simulink model "wahadlo3"  (R2018a)
settings: Solver=VariableStepAuto  StartTime=0.0  StopTime=100.0  RelTol=1e-3
settings Model: Creator=Koala  LastModifiedBy=Koala

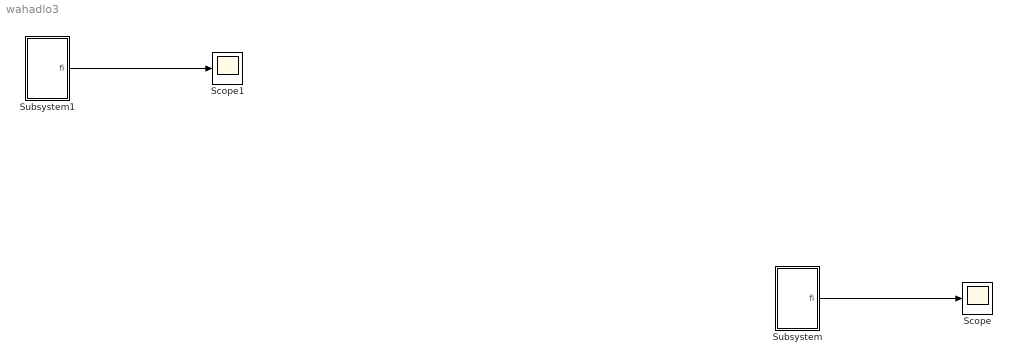
== system wahadlo3 ==
  Scope : Scope
  Scope1 : Scope
  Subsystem : Subsystem  mask{m=10, l=3, k=1, g=10, fi0=90}
      mask prompts: m "Masa"; l "Długość"; k "Tłumienie"; g "Przyśpieszenie"; fi0 "Kąt początkowy"
  Subsystem1 : Subsystem  mask{m=10, l=3, k=1, g=10, fi0=90}
      mask prompts: m "Masa"; l "Długość"; k "Tłumienie"; g "Przyśpieszenie"; fi0 "Kąt początkowy"
  wires:
  Subsystem/1(fi) -> Scope/1
  Subsystem1/1(fi) -> Scope1/1

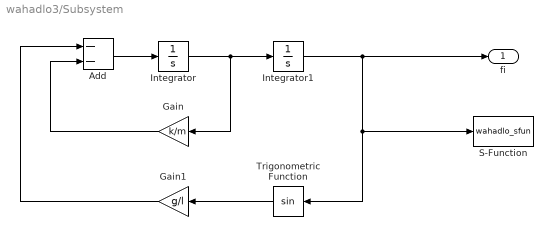
== system wahadlo3/Subsystem ==
  Add : Sum  Inputs=--
  Gain : Gain  Gain=k/m
  Gain1 : Gain  Gain=g/l
  Integrator : Integrator
  Integrator1 : Integrator  InitialCondition=fi0 * pi/180
  S-Function : S-Function  FunctionName=wahadlo_sfun  Parameters=l,m,fi0  SFunctionDeploymentMode=off  EnableBusSupport=off
  Trigonometric Function : Trigonometry
  fi : Outport
  wires:
  Integrator1/1 -> fi/1, S-Function/1, Trigonometric Function/1
  Integrator/1 -> Gain/1, Integrator1/1
  Gain1/1 -> Add/1
  Add/1 -> Integrator/1
  Gain/1 -> Add/2
  Trigonometric Function/1 -> Gain1/1

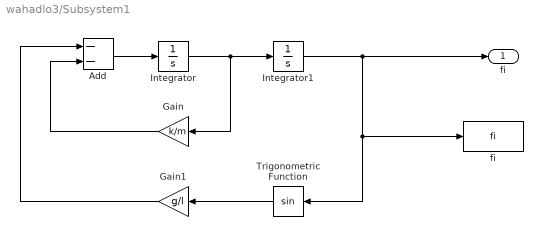
== system wahadlo3/Subsystem1 ==
  Add : Sum  Inputs=--
  Gain : Gain  Gain=k/m
  Gain1 : Gain  Gain=g/l
  Integrator : Integrator
  Integrator1 : Integrator  InitialCondition=fi0 * pi/180
  Trigonometric Function : Trigonometry
  "fi " : ToWorkspace  VariableName=fi  SampleTime=-1
  fi : Outport
  wires:
  Integrator1/1 -> fi/1, "fi "/1, Trigonometric Function/1
  Integrator/1 -> Gain/1, Integrator1/1
  Gain1/1 -> Add/1
  Add/1 -> Integrator/1
  Gain/1 -> Add/2
  Trigonometric Function/1 -> Gain1/1
